simulink model "root_locus_sim_example_1"  (Simulink 10.1)
settings: Solver=FixedStepAuto  StartTime=0.0  StopTime=stopTime  FixedStep=T  RelTol=1e-3
values from neighbouring files (symbols this model uses):
  A = [0, 1, 0; 0, 0, 1; 0, -2, -3]    [root_locus_example_1.m]
  B = [0;0;1]    [root_locus_example_1.m]
  C = [1 0 0]    [root_locus_example_1.m]
  d = [1, 3, 2]    [root_locus_example_2.m]
  n = [0, 0, 1]    [root_locus_example_2.m]
undefined symbols (not defined in the file or in its folder): K
settings Model: Creator=TULPAR  LastModifiedBy=TULPAR
settings DataIOCC: SaveFormat=Dataset  SaveTime=off  ReturnWorkspaceOutputs=on
settings OptimizationCC: LifeSpan=auto
settings DebuggingCC: UnderspecifiedInitializationDetection=Simplified  MergeDetectMultiDrivingBlocksExec=error  SFUnexpectedBacktrackingDiag=error  SFNoUnconditionalDefaultTransitionDiag=error  SFExecutionAtInitializationDiag=warning  ArithmeticOperatorsInVariantConditions=error
settings HardwareCC: ProdBitPerPointer=64  ProdBitPerSizeT=64  ProdBitPerPtrDiffT=64  ProdLargestAtomicFloat=Float  ProdIntDivRoundTo=Zero  ProdEndianess=LittleEndian  ProdWordSize=64  ProdHWDeviceType=Intel->x86-64 (Windows64)
settings ModelReferenceCC: PropagateSignalLabelsOutOfModel=on
settings SFSimCC: SimUseLocalCustomCode=on  CustomCodeUndefinedFunction=FilterOut
settings RTWCC: RTWUseLocalCustomCode=on
settings CodeAppCC: StateflowObjectComments=off
settings GRTTargetCC: TargetLangStandard=C99 (ISO)  CombineOutputUpdateFcns=on  GRTInterface=off
settings ConfigComp: CovMetricSettings=dwe  CovHtmlReporting=off  CovSaveCumulativeToWorkspaceVar=off  CovSaveSingleToWorkspaceVar=off  CovExternalEMLEnable=on

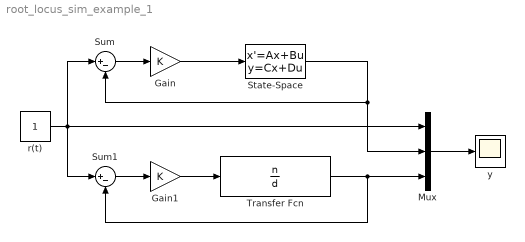
== system root_locus_sim_example_1 ==
  Gain : Gain  Gain=K
  Gain1 : Gain  Gain=K
  Mux : Mux  Inputs=3
  State-Space : StateSpace  A=A  B=B  C=C  D=0  InitialCondition=0
  Sum : Sum  Inputs=|+-
  Sum1 : Sum  Inputs=|+-
  Transfer Fcn : TransferFcn  Numerator=n  Denominator=d
  r(t) : Constant
  y : Scope
  wires:
  r(t)/1 -> Sum/1, Sum1/1, Mux/1
  Sum/1 -> Gain/1
  Gain/1 -> State-Space/1
  State-Space/1 -> Sum/2, Mux/2
  Sum1/1 -> Gain1/1
  Gain1/1 -> Transfer Fcn/1
  Transfer Fcn/1 -> Sum1/2, Mux/3
  Mux/1 -> y/1
